simulink model "ModelInvertedPD_Plant"  (R2022b)
settings: Solver=ode45  StartTime=0.0  StopTime=200.0  RelTol=1e-3  EnableMultiTasking=on
undefined symbols (not defined in the file): magnitude
settings Model: Creator=hp  LastModifiedBy=hp
settings SolverCC: AlgebraicLoopSolver=TrustRegion
settings DataIOCC: LimitDataPoints=on  SaveFormat=Array  SignalLoggingSaveFormat=ModelDataLogs  ReturnWorkspaceOutputs=off
settings OptimizationCC: InitFltsAndDblsToZero=on  LifeSpan=inf
settings DebuggingCC: SaveWithParameterizedLinksMsg=none  UnderspecifiedInitializationDetection=Classic  MergeDetectMultiDrivingBlocksExec=none  SignalResolutionControl=TryResolveAllWithWarning  SolverPrmCheckMsg=warning  MultiTaskDSMMsg=warning  MultiTaskCondExecSysMsg=none  FcnCallInpInsideContextMsg=warning  UnconnectedInputMsg=warning  UnconnectedOutputMsg=warning  UnconnectedLineMsg=warning  SFUnexpectedBacktrackingDiag=warning  SFNoUnconditionalDefaultTransitionDiag=warning  SFExecutionAtInitializationDiag=none  SFMachineParentedDataDiag=warning  ArithmeticOperatorsInVariantConditions=warning
settings HardwareCC: ProdBitPerPointer=32  ProdBitPerSizeT=32  ProdBitPerPtrDiffT=32  ProdLargestAtomicFloat=None  ProdIntDivRoundTo=Undefined  ProdEndianess=Unspecified  ProdWordSize=32  ProdHWDeviceType=32-bit Generic
settings ModelReferenceCC: PropagateSignalLabelsOutOfModel=off
settings CodeAppCC: StateflowObjectComments=on
settings GRTTargetCC: TargetFcnLib=ansi_tfl_tmw.mat  TargetLangStandard=C89/C90 (ANSI)  CombineOutputUpdateFcns=off  GRTInterface=on
settings ConfigComp: CovMetricSettings=dw  CovSaveCumulativeToWorkspaceVar=on  CovSaveSingleToWorkspaceVar=on

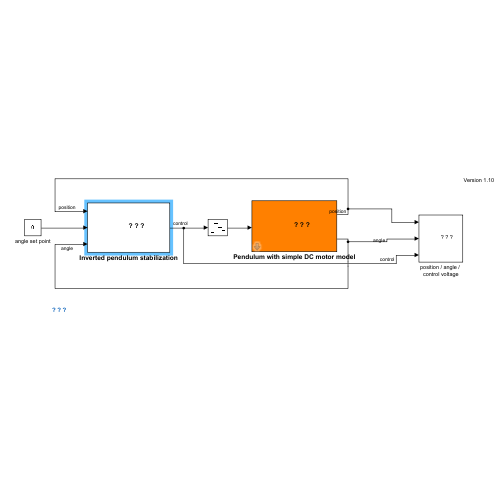
[thumbnail: Simulink's stored preview of the top-level diagram]
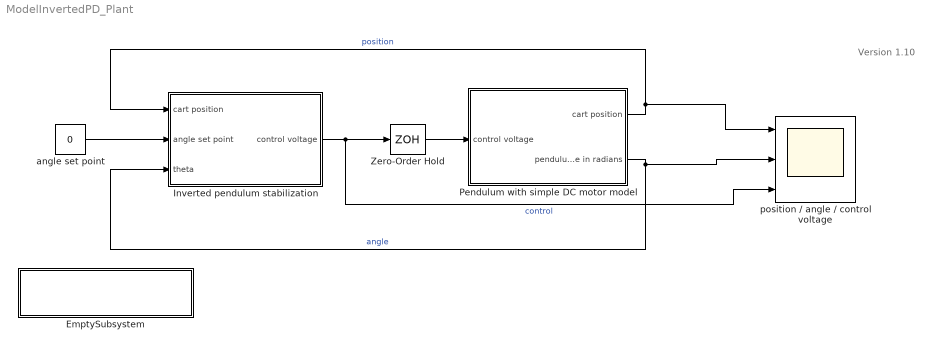
== system ModelInvertedPD_Plant ==
  note: Version 1.10
  EmptySubsystem : Subsystem
      mask Display:
      | image(imread('FB-inst-blue2.jpg'))
      | disp('\n\nFeedback Instruments Limited')
  Inverted pendulum stabilization : Subsystem
      mask Display: image(imread('bckg.bmp'))disp('Inverted pendulum \nstabilization')
  Pendulum with simple DC motor model : Subsystem  mask{m=0.23, cM=2.4, L=0.4, g=9.81, I=0.099, theta0=0.2, cart_friction=0.05, pend_damp=0.005}
      mask prompts: m "Pendulum mass"; cM "Cart mass"; L "Pendulum length"; g "gravitational constant"; I "Moment of inertia of the pole itself"; theta0 "Initial pendulum angle"; cart_friction "Cart friction coefficient"; pend_damp "Pendulum damping coefficient"
      mask Display: image(imread('pend.bmp'))
  Zero-Order Hold : ZeroOrderHold  SampleTime=0.001
  angle set point : Constant  Value=0
  position / angle / control voltage : Scope  NumInputPorts=3
      mask Display: image(imread('scope.jpg'))
  wires:
  Pendulum with simple DC motor model/1(cart position) -> Inverted pendulum stabilization/1(cart position), position / angle / control voltage/1  "position"
  Pendulum with simple DC motor model/2(pendulum angle in radians) -> Inverted pendulum stabilization/3(theta), position / angle / control voltage/2  "angle"
  angle set point/1 -> Inverted pendulum stabilization/2(angle set point)
  Inverted pendulum stabilization/1(control voltage) -> Zero-Order Hold/1, position / angle / control voltage/3  "control"
  Zero-Order Hold/1 -> Pendulum with simple DC motor model/1(control voltage)

== system ModelInvertedPD_Plant/EmptySubsystem ==

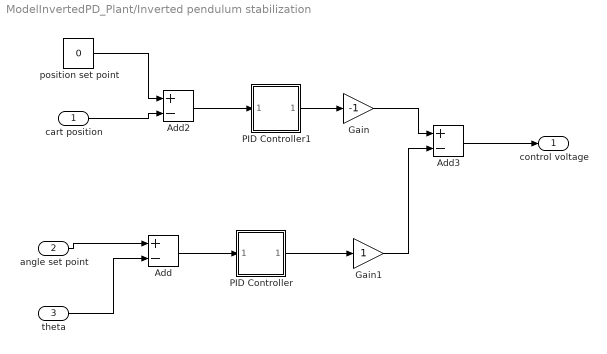
== system ModelInvertedPD_Plant/Inverted pendulum stabilization ==
  cart position : Inport
  angle set point : Inport  Port=2
  theta : Inport  Port=3
  Add : Sum  Inputs=+-
  Add2 : Sum  Inputs=+-
  Add3 : Sum  Inputs=+-
  Gain : Gain  Gain=-1
  Gain1 : Gain
  PID Controller : Subsystem  AncestorBlock=simulink_extras/Additional Linear/PID Controller  mask(PID Controller){P=40, I=5, D=9}
      mask prompts: P "Proportional:"; I "Integral:"; D "Derivative:"
      mask help:
      | Enter expressions for proportional, integral, and derivative terms.
      | P+I/s+Ds
      settings: LibrarySourceBlock=|
      | simulink_extras/Additional
      | Linear/PID Controller
      mask Help: This block implements a PID controller where parameters are entered for the Proportional, Integral and Derivative terms. Unmask this block to see how it works. The derivative term is implemented using a true derivative block.
      mask Display: image(imread('bckg.bmp'))disp('PID')
  PID Controller1 : Subsystem  AncestorBlock=simulink_extras/Additional Linear/PID Controller  mask(PID Controller){P=0.2, I=0.001, D=0}
      mask prompts: P "Proportional:"; I "Integral:"; D "Derivative:"
      mask help:
      | Enter expressions for proportional, integral, and derivative terms.
      | P+I/s+Ds
      settings: LibrarySourceBlock=|
      | simulink_extras/Additional
      | Linear/PID Controller
      mask Help: This block implements a PID controller where parameters are entered for the Proportional, Integral and Derivative terms. Unmask this block to see how it works. The derivative term is implemented using a true derivative block.
      mask Display: image(imread('bckg.bmp'))disp('PID')
  position set point : Constant  Value=0
  control voltage : Outport
  wires:
  PID Controller/1(Out_1) -> Gain1/1
  Add/1 -> PID Controller/1(In_1)
  position set point/1 -> Add2/1
  Add2/1 -> PID Controller1/1(In_1)
  PID Controller1/1(Out_1) -> Gain/1
  Gain/1 -> Add3/1
  cart position/1 -> Add2/2
  theta/1 -> Add/2
  angle set point/1 -> Add/1
  Add3/1 -> control voltage/1
  Gain1/1 -> Add3/2

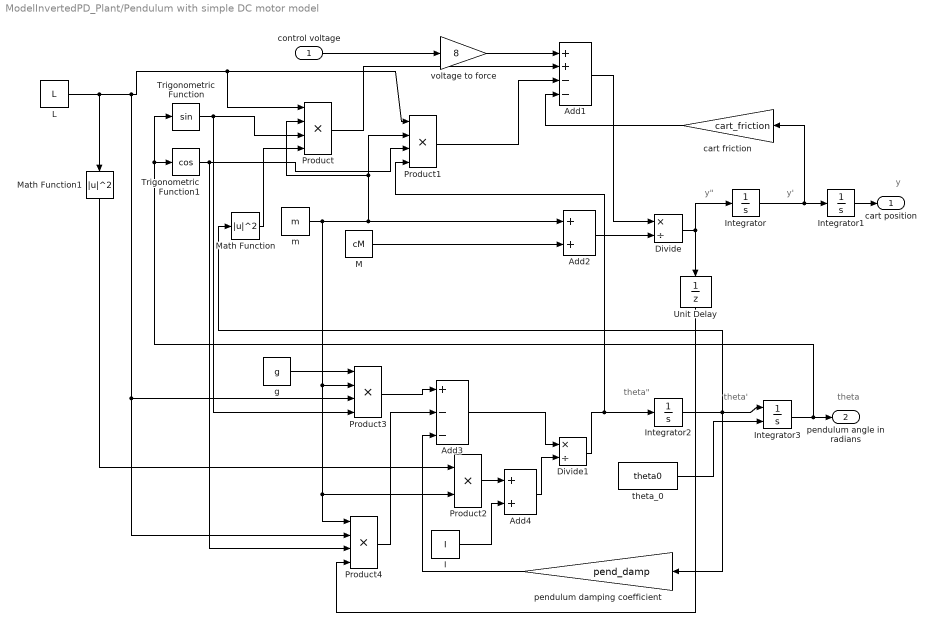
== system ModelInvertedPD_Plant/Pendulum with simple DC motor model ==
  note: y"
  note: y'
  note: theta"
  note: theta'
  note: theta
  note: y
  control voltage : Inport
  Add1 : Sum  Inputs=++--
  Add2 : Sum
  Add3 : Sum  Inputs=+--
  Add4 : Sum
  Divide : Product  Inputs=*/
  Divide1 : Product  Inputs=*/
  I : Constant  Value=I
  Integrator : Integrator
  Integrator1 : Integrator
  Integrator2 : Integrator
  Integrator3 : Integrator  InitialConditionSource=external
  L : Constant  Value=L
  M : Constant  Value=cM
  Math Function : Math  Operator=magnitude^2  SignedPower=on
  Math Function1 : Math  Operator=magnitude^2  SignedPower=on
  Product{,1,3..4} (4 alike) : Product  Inputs=4  RndMeth=Zero
  Product2 : Product  RndMeth=Zero
  Trigonometric Function : Trigonometry
  Trigonometric Function1 : Trigonometry  Operator=cos
  Unit Delay : UnitDelay  SampleTime=0.001
  cart friction : Gain  Gain=cart_friction
  g : Constant  Value=g
  m : Constant  Value=m
  pendulum damping coefficient : Gain  Gain=pend_damp
  theta_0 : Constant  Value=theta0
  voltage to force : Gain  Gain=8
  cart position : Outport
  pendulum angle in radians : Outport  Port=2
  wires:
  Unit Delay/1 -> Product4/4
  voltage to force/1 -> Add1/1
  I/1 -> Add4/2
  Add4/1 -> Divide1/2
  Product2/1 -> Add4/1
  Integrator1/1 -> cart position/1
  control voltage/1 -> voltage to force/1
  pendulum damping coefficient/1 -> Add3/3
  cart friction/1 -> Add1/4
  g/1 -> Product3/1
  Product4/1 -> Add3/2
  Product3/1 -> Add3/1
  Math Function1/1 -> Product2/1
  Add3/1 -> Divide1/1
  Trigonometric Function1/1 -> Product4/3, Product1/3
  Product1/1 -> Add1/3
  Product/1 -> Add1/2
  Math Function/1 -> Product/4
  theta_0/1 -> Integrator3/2
  Trigonometric Function/1 -> Product3/4, Product/3
  L/1 -> Product4/2, Product3/3, Product1/1, Product/1, Math Function1/1
  Divide1/1 -> Product1/4, Integrator2/1
  Divide/1 -> Unit Delay/1, Integrator/1
  Add1/1 -> Divide/1
  Add2/1 -> Divide/2
  M/1 -> Add2/2
  m/1 -> Product4/1, Product2/2, Product3/2, Product1/2, Product/2, Add2/1
  Integrator3/1 -> pendulum angle in radians/1, Trigonometric Function/1, Trigonometric Function1/1
  Integrator2/1 -> pendulum damping coefficient/1, Math Function/1, Integrator3/1
  Integrator/1 -> cart friction/1, Integrator1/1

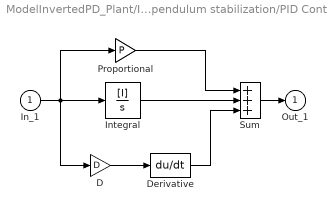
== system ModelInvertedPD_Plant/Inverted pendulum stabilization/PID Controller ==
  In_1 : Inport
  D : Gain  Gain=D  SaturateOnIntegerOverflow=on  OutDataTypeStr=Inherit: Same as input  ParamDataTypeStr=Inherit: Same as input
  Derivative : Derivative
  Integral : TransferFcn  Numerator=[I]  Denominator=[1 0]
  Proportional : Gain  Gain=P  SaturateOnIntegerOverflow=on  OutDataTypeStr=Inherit: Same as input  ParamDataTypeStr=Inherit: Same as input
  Sum : Sum  Inputs=+++  InputSameDT=on  SaturateOnIntegerOverflow=on  OutDataTypeStr=Inherit: Same as first input
  Out_1 : Outport  InitialOutput=0
  wires:
  Proportional/1 -> Sum/1
  Integral/1 -> Sum/2
  Derivative/1 -> Sum/3
  In_1/1 -> Integral/1, Proportional/1, D/1
  Sum/1 -> Out_1/1
  D/1 -> Derivative/1

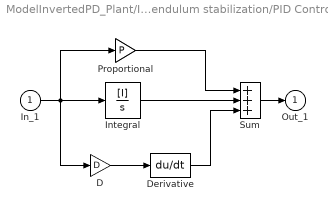
== system ModelInvertedPD_Plant/Inverted pendulum stabilization/PID Controller1 ==
  In_1 : Inport
  D : Gain  Gain=D  SaturateOnIntegerOverflow=on  OutDataTypeStr=Inherit: Same as input  ParamDataTypeStr=Inherit: Same as input
  Derivative : Derivative
  Integral : TransferFcn  Numerator=[I]  Denominator=[1 0]
  Proportional : Gain  Gain=P  SaturateOnIntegerOverflow=on  OutDataTypeStr=Inherit: Same as input  ParamDataTypeStr=Inherit: Same as input
  Sum : Sum  Inputs=+++  InputSameDT=on  SaturateOnIntegerOverflow=on  OutDataTypeStr=Inherit: Same as first input
  Out_1 : Outport  InitialOutput=0
  wires:
  Proportional/1 -> Sum/1
  Integral/1 -> Sum/2
  Derivative/1 -> Sum/3
  In_1/1 -> Integral/1, Proportional/1, D/1
  Sum/1 -> Out_1/1
  D/1 -> Derivative/1
